simulink model "controltest"  (R2021b)
settings: Solver=ode113  StartTime=0.0  StopTime=tfinal  MaxStep=tstepMax  RelTol=1e-4  AbsTol=1e-4
values from neighbouring files (symbols this model uses):
  a_b = 10    [Optimization.m]    (also in SI_Loop.m; simrun.m)
  damping = 0    [Optimization.m]    (also in SI_Loop.m; simrun.m)
  gainD = PIDvals(ic)    [Optimization.m]    (also in SI_Loop.m = 75; simrun.m = 10)
  gainI = PIDvals(ic)    [Optimization.m]    (also in SI_Loop.m = 0; simrun.m = 10)
  gainP = PIDvals(ic)    [Optimization.m]    (also in SI_Loop.m = 75; simrun.m = 100)
  k_m = k/m    [Optimization.m]    (also in SI_Loop.m = 0; simrun.m = 8)
  R_0 = 2    [Optimization.m]    (also in SI_Loop.m = 2000; simrun.m)
  rate_pre = 2*pi/T    [Optimization.m]    (also in SI_Loop.m; simrun.m)
  theta0 = 0    [Optimization.m]    (also in RotatingSpring.m; RotatingSpringFeedback.m; SI_Loop.m; rotatingSpringLoop.m)
  thetadot0 = 40    [Optimization.m]    (also in RotatingSpring.m = 10; RotatingSpringFeedback.m = 10; SI_Loop.m = 0.012301296218; rotatingSpringLoop.m = thetadot0vals(i))
  x0 = 0    [Optimization.m]    (also in RotatingSpring.m; RotatingSpringFeedback.m; SI_Loop.m; simEom.m)
  xdot0 = 0    [Optimization.m]    (also in RotatingSpring.m; RotatingSpringFeedback.m; SI_Loop.m; simEom.m)
libraries: slpidlib x1
settings Model: Creator=alexandermayo-smith  LastModifiedBy=alexandermayo-smith
settings SolverCC: ShapePreserveControl=EnableAll

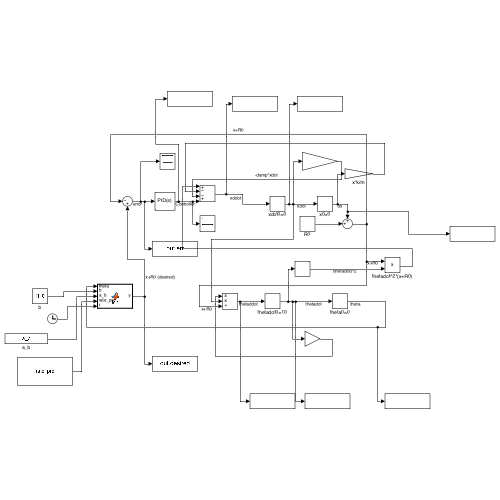
[thumbnail: Simulink's stored preview of the top-level diagram]
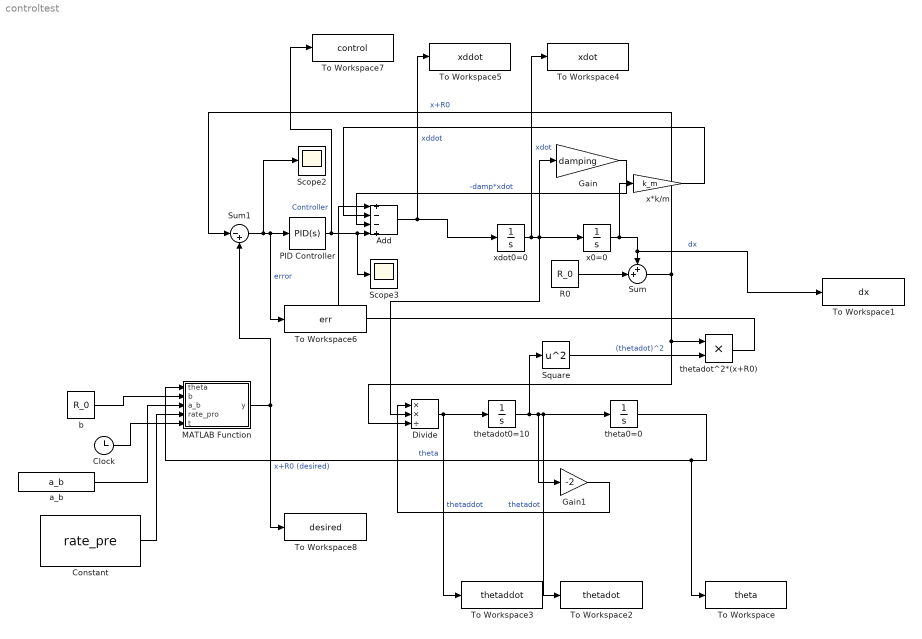
== system controltest ==
  Add : Sum  Inputs=+--+
  Clock : Clock
  Constant : Constant  Value=rate_pre
  Divide : Product  Inputs=**/
  Gain : Gain  Gain=damping
  Gain1 : Gain  Gain=-2
  MATLAB Function : MATLAB Function  TreatAsAtomicUnit=on
  PID Controller : slpidlib/PID Controller  Controller=PID  Form=Parallel  TimeDomain=Continuous-time  UseExternalTs=off  SampleTime=-1  IntegratorMethod=Forward Euler  FilterMethod=Forward Euler  ControllerParametersSource=internal  P=gainP  I=gainI  D=gainD  UseFilter=on  N=100  TunerSelectOption=Transfer Function Based (PID Tuner App)  InitialConditionSource=internal  InitialConditionForIntegrator=0  InitialConditionForFilter=0  DifferentiatorICPrevScaledInput=0  ExternalReset=none  TrackingMode=off  Kt=1  LimitOutput=off  SatLimitsSource=internal  UpperSaturationLimit=inf  LowerSaturationLimit=-inf  LinearizeAsGain=on  AntiWindupMode=none  Kb=1  POutMin=[]  POutMax=[]  IOutMin=[]  IOutMax=[]  DOutMin=[]  DOutMax=[]  NOutMin=[]  NOutMax=[]  SumOutMin=[]  SumOutMax=[]  SaturationOutMin=[]  SaturationOutMax=[]  PParamMin=[]  PParamMax=[]  IParamMin=[]  IParamMax=[]  DParamMin=[]  DParamMax=[]  NParamMin=[]  NParamMax=[]  KbParamMin=[]  KbParamMax=[]  KtParamMin=[]  KtParamMax=[]  KbOutMin=[]  KbOutMax=[]  KtOutMin=[]  KtOutMax=[]  IntegratorOutMin=[]  IntegratorOutMax=[]  FilterOutMin=[]  FilterOutMax=[]  SumI1OutMin=[]  SumI1OutMax=[]  SumI2OutMin=[]  SumI2OutMax=[]  SumI3OutMin=[]  SumI3OutMax=[]  SumI4OutMin=[]  SumI4OutMax=[]  SumDOutMin=[]  SumDOutMax=[]  DifferentiatorOutMin=[]  DifferentiatorOutMax=[]  FilterDiffOutCoefMin=[]  FilterDiffOutCoefMax=[]  ReciprocalOutMin=[]  ReciprocalOutMax=[]  SumDenOutMin=[]  SumDenOutMax=[]  SumNumOutMin=[]  SumNumOutMax=[]  DivideOutMin=[]  DivideOutMax=[]  UdiffTsProdOutMin=[]  UdiffTsProdOutMax=[]  NTsProdOutMin=[]  NTsProdOutMax=[]  UintegralTsProdOutMin=[]  UintegralTsProdOutMax=[]  UngainTsProdOutMin=[]  UngainTsProdOutMax=[]  IntegratorContinuousStateAttributes=''  IntegratorStateMustResolveToSignalObject=off  IntegratorRTWStateStorageClass=Auto  FilterContinuousStateAttributes=''  FilterStateMustResolveToSignalObject=off  FilterRTWStateStorageClass=Auto  ParallelPVariant=InternalParameters  IdealPVariant=Disabled  IVariant=InternalParameters  DVariant=InternalParameters  IntegratorVariant=Continuous  SatVariant=Disabled  AWVariant=Passthrough  PCopyVariant=Disabled  TRVariant=Disabled  FdbkBlocksVariant=Forward  IdealPFdbkVariant=Disabled  SatFdbkVariant=Disabled  DerivativeFilterVariant=ContFilter  NVariant=InternalParameters  NCopyVariant=Disabled  FilterICVariant=InternalICsFilter  IntegratorICVariant=InternalICs  ExternalResetVariant=Disabled  TRSumVariant=Passthrough  SumFdbkVariant=Disabled  SumVariant=Sum_PID  TsampFilterVariant=InternalTs  TsampNgainVariant=Passthrough  TsampIntegralVariant=Passthrough  ExternalSaturationOutDataTypeStr=Inherit: Same as second input
  R0 : Constant  Value=R_0
  Scope2 : Scope
  Scope3 : Scope
  Square : Math  Operator=square  SaturateOnIntegerOverflow=on
  Sum : Sum  Inputs=++|
  Sum1 : Sum  Inputs=|-+
  To Workspace : ToWorkspace  VariableName=theta  SampleTime=-1
  To Workspace1 : ToWorkspace  VariableName=dx  SampleTime=-1
  To Workspace2 : ToWorkspace  VariableName=thetadot  SampleTime=-1
  To Workspace3 : ToWorkspace  VariableName=thetaddot  SampleTime=-1
  To Workspace4 : ToWorkspace  VariableName=xdot  SampleTime=-1
  To Workspace5 : ToWorkspace  VariableName=xddot  SampleTime=-1
  To Workspace6 : ToWorkspace  VariableName=err  SampleTime=-1
  To Workspace7 : ToWorkspace  VariableName=control  SampleTime=-1
  To Workspace8 : ToWorkspace  VariableName=desired  SampleTime=-1
  a_b : Constant  Value=a_b
  b : Constant  Value=R_0
  theta0=0 : Integrator  InitialCondition=theta0
  thetadot0=10 : Integrator  InitialCondition=thetadot0
  thetadot^2*(x+R0) : Product
  x*k/m : Gain  Gain=k_m
  x0=0 : Integrator  InitialCondition=x0
  xdot0=0 : Integrator  InitialCondition=xdot0
  wires:
  Divide/1 -> To Workspace3/1, thetadot0=10/1  "thetaddot"
  thetadot0=10/1 -> Square/1, Gain1/1, theta0=0/1, To Workspace2/1  "thetadot"
  Add/1 -> To Workspace5/1, xdot0=0/1  "xddot"
  xdot0=0/1 -> To Workspace4/1, Divide/2, Gain/1, x0=0/1  "xdot"
  x0=0/1 -> x*k/m/1, To Workspace1/1, Sum/1  "dx"
  Square/1 -> thetadot^2*(x+R0)/2  "(thetadot)^2"
  R0/1 -> Sum/2
  Sum/1 -> Divide/3, thetadot^2*(x+R0)/1, Sum1/1  "x+R0"
  thetadot^2*(x+R0)/1 -> Add/1
  Gain/1 -> Add/3  "-damp*xdot"
  Gain1/1 -> Divide/1
  PID Controller/1 -> To Workspace7/1, Scope3/1, Add/4  "Controller"
  Sum1/1 -> Scope2/1, To Workspace6/1, PID Controller/1  "error"
  a_b/1 -> MATLAB Function/3(a_b)
  b/1 -> MATLAB Function/2(b)
  x*k/m/1 -> Add/2
  MATLAB Function/1(y) -> To Workspace8/1, Sum1/2  "x+R0 (desired)"
  theta0=0/1 -> To Workspace/1, MATLAB Function/1(theta)  "theta"
  Clock/1 -> MATLAB Function/5(t)
  Constant/1 -> MATLAB Function/4(rate_pro)

== matlab function controltest/MATLAB Function ==
  data: theta input; y output; b input; a_b input; rate_pro input; t input
function y = fcn(theta, b, a_b,rate_pro,t)

a=b*a_b;
thetadisp=rate_pro*t;
y=(a*b)/(sqrt(b^2*sin(theta+thetadisp)^2 + a^2*cos(theta+thetadisp)^2));
